simulink model "AM_coherent_2020"  (R2020a)
settings: Solver=ode45  StartTime=0.0  StopTime=30  RelTol=1e-3  EnableMultiTasking=on
libraries: dsparch4 x3
settings Model: Creator=morelos_zaragoza  LastModifiedBy=000098944
settings DataIOCC: LimitDataPoints=on  SaveFormat=Array  SignalLoggingSaveFormat=ModelDataLogs  ReturnWorkspaceOutputs=off
settings OptimizationCC: ExpressionDepthLimit=2147483647  InitFltsAndDblsToZero=on  LifeSpan=inf
settings DebuggingCC: SaveWithParameterizedLinksMsg=none  UnderspecifiedInitializationDetection=Classic  MergeDetectMultiDrivingBlocksExec=none  SignalResolutionControl=TryResolveAllWithWarning  SolverPrmCheckMsg=warning  MultiTaskDSMMsg=warning  MultiTaskCondExecSysMsg=none  FcnCallInpInsideContextMsg=warning  StateNameClashWarn=warning  SFUnexpectedBacktrackingDiag=warning  SFNoUnconditionalDefaultTransitionDiag=warning  SFExecutionAtInitializationDiag=none  ArithmeticOperatorsInVariantConditions=warning
settings HardwareCC: ProdBitPerPointer=32  ProdBitPerSizeT=32  ProdBitPerPtrDiffT=32  ProdLargestAtomicFloat=None  ProdIntDivRoundTo=Undefined  ProdEndianess=Unspecified  ProdWordSize=32  ProdHWDeviceType=32-bit Generic
settings ModelReferenceCC: PropagateSignalLabelsOutOfModel=off
settings SFSimCC: SimUseLocalCustomCode=off  CustomCodeUndefinedFunction=UseInterfaceOnly
settings RTWCC: RTWUseLocalCustomCode=off
settings CodeAppCC: StateflowObjectComments=on
settings GRTTargetCC: TargetFcnLib=ansi_tfl_tmw.mat  TargetLangStandard=C89/C90 (ANSI)  CombineOutputUpdateFcns=off  GRTInterface=on
settings ConfigComp: CovMetricSettings=dw  CovHtmlReporting=on  CovSaveCumulativeToWorkspaceVar=on  CovSaveSingleToWorkspaceVar=on  CovExternalEMLEnable=off

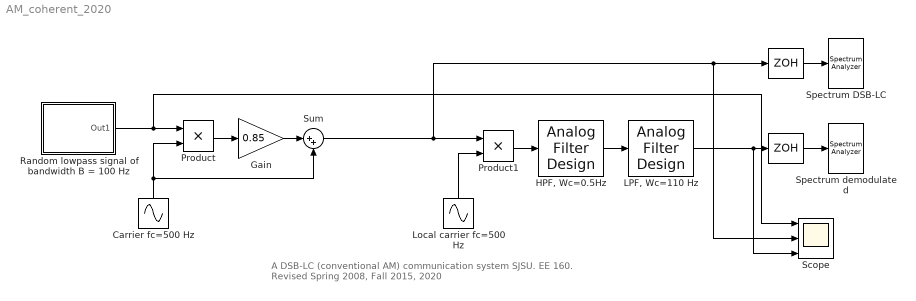
== system AM_coherent_2020 ==
  note: A DSB-LC (conventional AM) communication system
      | SJSU. EE 160. Revised Spring 2008, Fall 2015, 2020
  "  " : ZeroOrderHold  SampleTime=1/(25*90)
  "   " : ZeroOrderHold  SampleTime=1/(25*90)
  "   Carrier fc=500 Hz" : Sin  Frequency=2*pi*500  SampleTime=0
  Gain : Gain  Gain=0.85
  "HPF, Wc=0.5Hz" : dsparch4/Analog Filter Design  method=Butterworth  filttype=Highpass  N=4  Wlo=2*pi*0.5  Whi=2*pi*110  Rp=2  Rs=40
  "LPF, Wc=110 Hz" : dsparch4/Analog Filter Design  method=Butterworth  filttype=Lowpass  N=4  Wlo=2*pi*110  Whi=2*pi*110  Rp=2  Rs=40
  Local carrier fc=500 Hz : Sin  Frequency=2*pi*500  SampleTime=0
  Product : Product  RndMeth=Zero
  Product1 : Product  RndMeth=Zero
  Random lowpass signal of bandwidth B = 100 Hz : Subsystem  TreatAsAtomicUnit=on
  Scope : Scope  NumInputPorts=3
  Spectrum DSB-LC : SpectrumAnalyzer
  Spectrum demodulated : SpectrumAnalyzer
  Sum : Sum  Inputs=|++
  wires:
  Random lowpass signal of bandwidth B = 100 Hz/1(Out1) -> Product/1, Scope/1
  "   Carrier fc=500 Hz"/1 -> Product/2, Sum/2
  "  "/1 -> Spectrum DSB-LC/1
  "   "/1 -> Spectrum demodulated/1
  "LPF, Wc=110 Hz"/1 -> "   "/1, Scope/3
  Product/1 -> Gain/1
  Sum/1 -> "  "/1, Scope/2, Product1/1
  "HPF, Wc=0.5Hz"/1 -> "LPF, Wc=110 Hz"/1
  Local carrier fc=500 Hz/1 -> Product1/2
  Product1/1 -> "HPF, Wc=0.5Hz"/1
  Gain/1 -> Sum/1

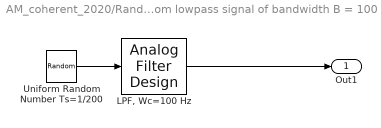
== system AM_coherent_2020/Random lowpass signal of bandwidth B = 100 Hz ==
  "LPF, Wc=100 Hz" : dsparch4/Analog Filter Design  method=Butterworth  filttype=Lowpass  N=22  Wlo=2*pi*100  Whi=2*pi*110  Rp=2  Rs=40
  Uniform Random Number Ts=1/200 : UniformRandomNumber  Seed=23453  SampleTime=1/200
  Out1 : Outport
  wires:
  Uniform Random Number Ts=1/200/1 -> "LPF, Wc=100 Hz"/1
  "LPF, Wc=100 Hz"/1 -> Out1/1
